simulink model "Stateflows"  (R2020a)
settings: Solver=FixedStepAuto  StartTime=0.0  StopTime=10.0  FixedStep=1e-3  RelTol=1e-3  EnableMultiTasking=on
undefined symbols (not defined in the file): D0, D1, D10, D11, D12, D13, D2, D3, D4, D5, D6, D7, D8, D9, PTA0, PTA1, PTA2, PTB23, PTB9, PTC16, PTC17, PTC2, PTC3, PTC4, PTD0, PTD1, PTD2, PTD3
libraries: frdmk64flib x17
settings Model: ExtModeTrigDuration=5  Creator=Luis  LastModifiedBy=jordanbierbrier
settings OptimizationCC: EnhancedBackFolding=on  PassReuseOutputArgsAs=Individual arguments  ZeroExternalMemoryAtStartup=off  ZeroInternalMemoryAtStartup=off  MaxStackSize=64  OptimizeBlockOrder=speed  DifferentSizesBufferReuse=on  OptimizationCustomize=off  EfficientTunableParamExpr=on
settings DebuggingCC: ParameterTunabilityLossMsg=error
settings HardwareCC: ProdBitPerPointer=32  ProdBitPerSizeT=32  ProdBitPerPtrDiffT=32  ProdLargestAtomicInteger=Long  ProdLargestAtomicFloat=Double  ProdWordSize=32  ProdHWDeviceType=ARM Compatible->ARM Cortex
settings SFSimCC: MATLABDynamicMemAlloc=off
settings RTWCC: SystemTargetFile=ert.tlc  HardwareBoard=NXP FRDM-K64F  TemplateMakefile=ert_default_tmf  Toolchain=GNU Tools for ARM Embedded Processors
settings CodeAppCC: ForceParamTrailComments=on  IgnoreCustomStorageClasses=off  OperatorAnnotations=on  SimulinkDataObjDesc=on  SFDataObjDesc=on  InsertBlockDesc=on

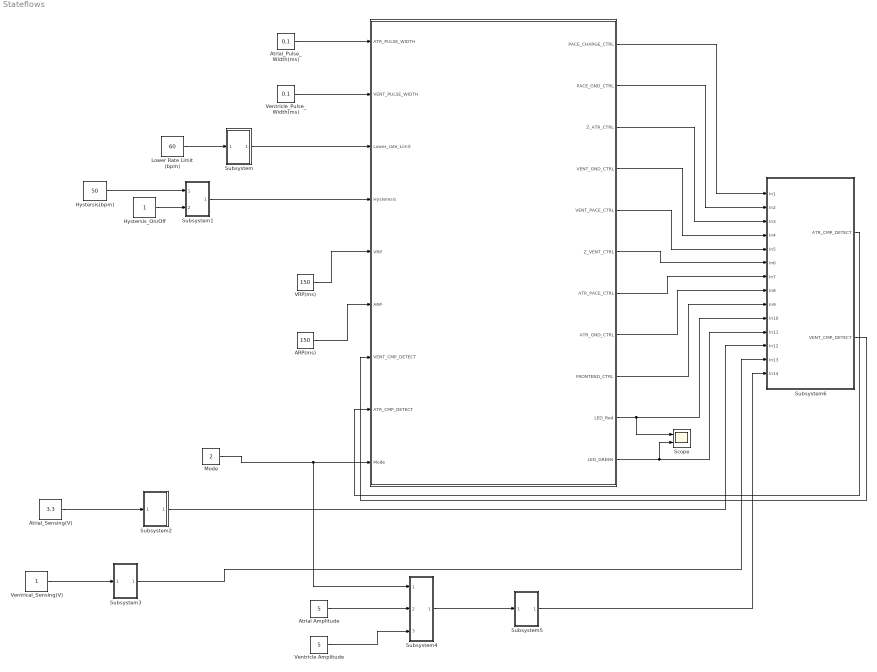
== system Stateflows ==
  " " : Stateflow chart  TreatAsAtomicUnit=on
      settings: PortSchema="{\"entries\":[{\"content\":{\"sides\":[{\"content\":{\"connectorIds\":[\"In1\",\"In4\",\"In2\",\"In9\",\"In5\",\"In6\",\"In7\",\"In8\",\"In3\"]},\"type\":\"ConnectorPlacement.EquallySpacedRectSide\",\"uuid\":\"f97b12ff-cb00-4386-a373-7143c3a8b48d\"},{\"content\":{\"connectorIds\":[\"Out1\",\"Out2\",\"Out3\",\"Out4\",\"Out5\",\"Out6\",\"Out7\",\"Out8\",\"Out9\",\"Out10\",\"Out11\"],\"side\":\"RIGHT\"},\"type\":\"ConnectorPlacement.EquallySpacedRectSide\",\"uuid\":\"90163773-f9d1-46de-bd72-9589b8539202\"},{\"content\":{\"connectorIds\":[],\"side\":\"TOP\"},\"type\":\"ConnectorPlacement.EquallySpacedRectSide\",\"uuid\":\"f8a54119-a7c4-4071-8260-df405210e670\"}]},\"type\":\"ConnectorPlacement.EquallySpacedConnector\",\"uuid\":\"47f7c40c-c42b-42f7-beed-99d299c6cdee\"}],\"packageUris\":[\"http://schema.mathworks.com/mf0/Connector/19700101\"],\"version\":\"1.0\"}"
  ARP(ms) : Constant  Value=150  OutDataTypeStr=uint16
  Atrial Amplitude : Constant  Value=5  OutDataTypeStr=double
  Atrial_Pulse_Width(ms) : Constant  Value=0.1  OutDataTypeStr=double
  Atrial_Sensing(V) : Constant  Value=3.3  OutDataTypeStr=double
  Hystersis(bpm) : Constant  Value=50  OutDataTypeStr=uint16
  Hystersis_On/Off : Constant  OutDataTypeStr=uint16
  Lower Rate Limit (bpm) : Constant  Value=60  OutDataTypeStr=uint16
  Mode : Constant  Value=2  OutDataTypeStr=uint8
  Scope : Scope  NumInputPorts=2
  Subsystem : Subsystem
  Subsystem1 : Subsystem
  Subsystem2 : Subsystem
  Subsystem3 : Subsystem
  Subsystem4 : Subsystem
  Subsystem5 : Subsystem
  Subsystem6 : Subsystem
  VRP(ms) : Constant  Value=150  OutDataTypeStr=uint16
  Ventrical_Sensing(V) : Constant  OutDataTypeStr=double
  Ventricle Amplitude : Constant  Value=5  OutDataTypeStr=double
  Ventricle_Pulse_Width(ms) : Constant  Value=0.1  OutDataTypeStr=double
  wires:
  Atrial_Pulse_Width(ms)/1 -> " "/1(ATR_PULSE_WIDTH)
  Mode/1 -> Subsystem4/1(In1), " "/3(Mode)
  Ventricle_Pulse_Width(ms)/1 -> " "/4(VENT_PULSE_WIDTH)
  ARP(ms)/1 -> " "/6(ARP)
  VRP(ms)/1 -> " "/5(VRP)
  Lower Rate Limit (bpm)/1 -> Subsystem/1(In1)
  Subsystem/1(Out1) -> " "/2(Lower_rate_Limit)
  Hystersis(bpm)/1 -> Subsystem1/1(In1)
  Hystersis_On/Off/1 -> Subsystem1/2(In2)
  Subsystem1/1(Out1) -> " "/9(Hysteresis)
  Atrial_Sensing(V)/1 -> Subsystem2/1(In1)
  Ventrical_Sensing(V)/1 -> Subsystem3/1(In1)
  Atrial Amplitude/1 -> Subsystem4/2(In2)
  Ventricle Amplitude/1 -> Subsystem4/3(In3)
  Subsystem4/1(Out1) -> Subsystem5/1(In1)
  " "/1(PACE_CHARGE_CTRL) -> Subsystem6/1(In1)
  " "/2(PACE_GND_CTRL) -> Subsystem6/2(In2)
  " "/3(Z_ATR_CTRL) -> Subsystem6/3(In3)
  " "/4(VENT_GND_CTRL) -> Subsystem6/4(In4)
  " "/5(VENT_PACE_CTRL) -> Subsystem6/5(In5)
  " "/6(Z_VENT_CTRL) -> Subsystem6/6(In6)
  " "/7(ATR_PACE_CTRL) -> Subsystem6/7(In7)
  " "/8(ATR_GND_CTRL) -> Subsystem6/8(In8)
  " "/9(FRONTEND_CTRL) -> Subsystem6/9(In9)
  " "/10(LED_Red) -> Scope/1, Subsystem6/10(In10)
  " "/11(LED_GREEN) -> Scope/2, Subsystem6/11(In11)
  Subsystem2/1(Out1) -> Subsystem6/12(In12)
  Subsystem3/1(Out1) -> Subsystem6/13(In13)
  Subsystem5/1(Out1) -> Subsystem6/14(In14)
  Subsystem6/1(ATR_CMP_DETECT) -> " "/8(ATR_CMP_DETECT)
  Subsystem6/2(VENT_CMP_DETECT) -> " "/7(VENT_CMP_DETECT)

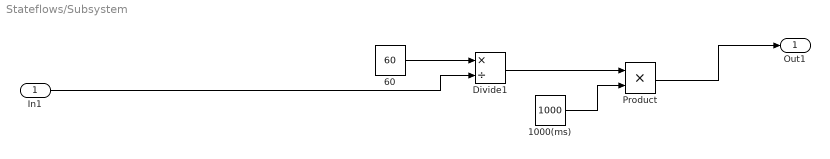
== system Stateflows/Subsystem ==
  In1 : Inport
  1000(ms) : Constant  Value=1000  OutDataTypeStr=uint16
  60 : Constant  Value=60  OutDataTypeStr=uint16
  Divide1 : Product  Inputs=*/
  Product : Product  OutDataTypeStr=uint16
  Out1 : Outport
  wires:
  60/1 -> Divide1/1
  In1/1 -> Divide1/2
  Product/1 -> Out1/1
  Divide1/1 -> Product/1
  1000(ms)/1 -> Product/2

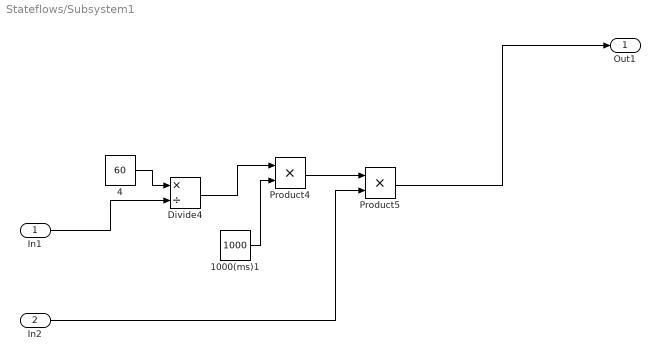
== system Stateflows/Subsystem1 ==
  In1 : Inport
  In2 : Inport  Port=2
  1000(ms)1 : Constant  Value=1000  OutDataTypeStr=uint16
  4 : Constant  Value=60  OutDataTypeStr=uint16
  Divide4 : Product  Inputs=*/
  Product4 : Product  OutDataTypeStr=uint16
  Product5 : Product  OutDataTypeStr=uint16
  Out1 : Outport
  wires:
  In2/1 -> Product5/2
  Product5/1 -> Out1/1
  Divide4/1 -> Product4/1
  Product4/1 -> Product5/1
  4/1 -> Divide4/1
  In1/1 -> Divide4/2
  1000(ms)1/1 -> Product4/2

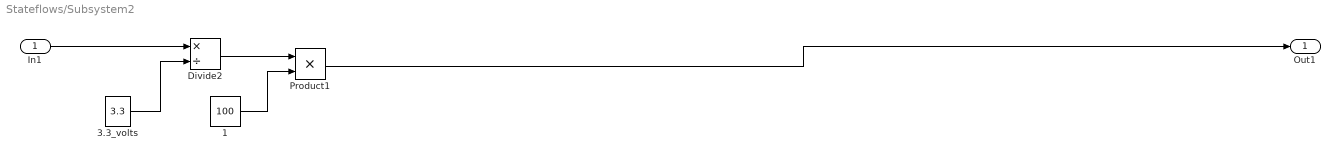
== system Stateflows/Subsystem2 ==
  In1 : Inport
  1 : Constant  Value=100  OutDataTypeStr=uint16
  3.3_volts : Constant  Value=3.3  OutDataTypeStr=double
  Divide2 : Product  Inputs=*/
  Product1 : Product  OutDataTypeStr=uint16
  Out1 : Outport
  wires:
  Product1/1 -> Out1/1
  1/1 -> Product1/2
  In1/1 -> Divide2/1
  Divide2/1 -> Product1/1
  3.3_volts/1 -> Divide2/2

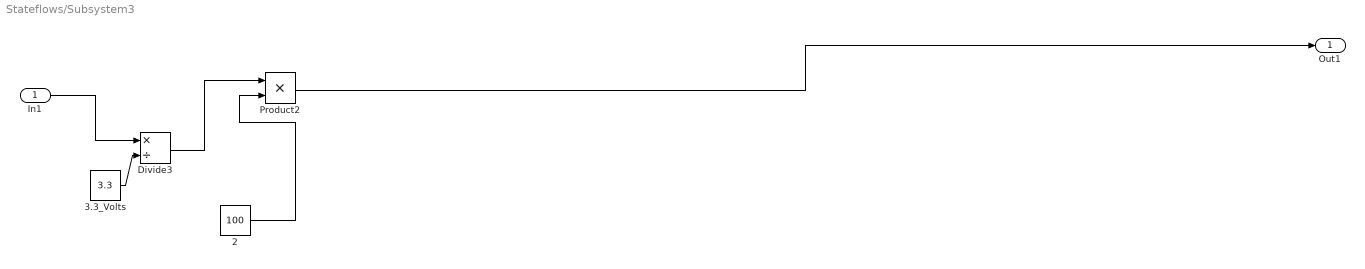
== system Stateflows/Subsystem3 ==
  In1 : Inport
  2 : Constant  Value=100  OutDataTypeStr=uint16
  3.3_Volts : Constant  Value=3.3  OutDataTypeStr=double
  Divide3 : Product  Inputs=*/
  Product2 : Product  OutDataTypeStr=uint16
  Out1 : Outport
  wires:
  Product2/1 -> Out1/1
  3.3_Volts/1 -> Divide3/2
  Divide3/1 -> Product2/1
  In1/1 -> Divide3/1
  2/1 -> Product2/2

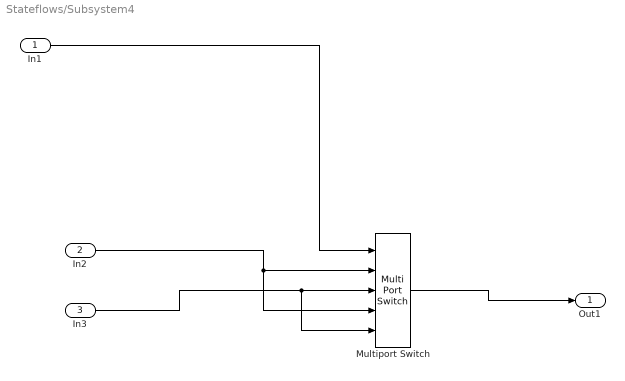
== system Stateflows/Subsystem4 ==
  In1 : Inport
  In2 : Inport  Port=2
  In3 : Inport  Port=3
  Multiport Switch : MultiPortSwitch  DataPortOrder=Zero-based contiguous  Inputs=4  zeroidx=on  OutDataTypeStr=double
  Out1 : Outport
  wires:
  Multiport Switch/1 -> Out1/1
  In3/1 -> Multiport Switch/5, Multiport Switch/3
  In1/1 -> Multiport Switch/1
  In2/1 -> Multiport Switch/4, Multiport Switch/2

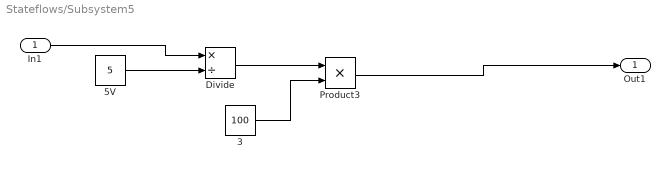
== system Stateflows/Subsystem5 ==
  In1 : Inport
  3 : Constant  Value=100  OutDataTypeStr=uint16
  5V : Constant  Value=5  OutDataTypeStr=uint16
  Divide : Product  Inputs=*/  OutDataTypeStr=uint16
  Product3 : Product  OutDataTypeStr=uint16
  Out1 : Outport
  wires:
  Product3/1 -> Out1/1
  3/1 -> Product3/2
  In1/1 -> Divide/1
  Divide/1 -> Product3/1
  5V/1 -> Divide/2

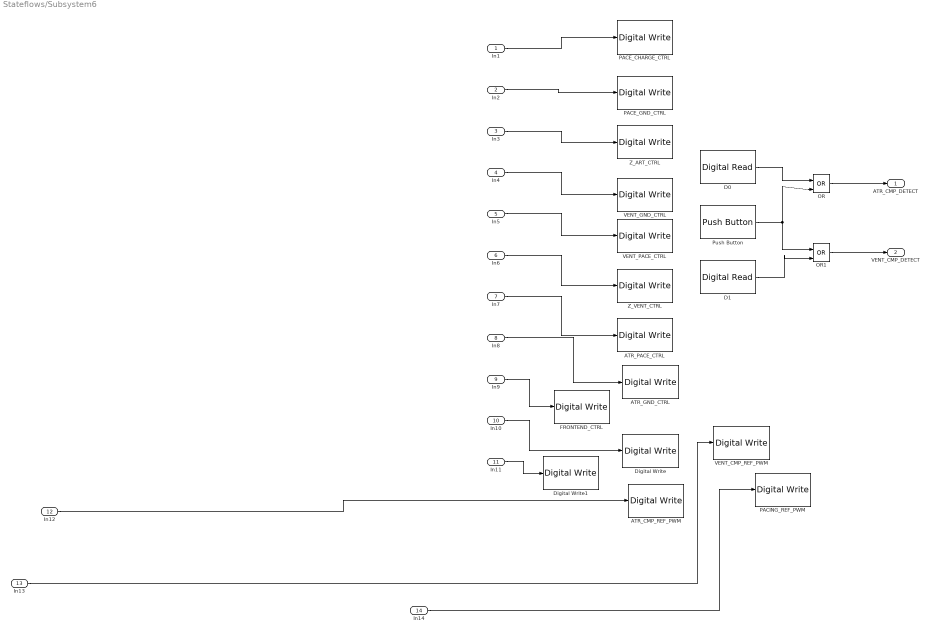
== system Stateflows/Subsystem6 ==
  In1 : Inport
  In2 : Inport  Port=2
  In3 : Inport  Port=3
  In4 : Inport  Port=4
  In5 : Inport  Port=5
  In6 : Inport  Port=6
  In7 : Inport  Port=7
  In8 : Inport  Port=8
  In9 : Inport  Port=9
  In10 : Inport  Port=10
  In11 : Inport  Port=11
  In12 : Inport  Port=12
  In13 : Inport  Port=13
  In14 : Inport  Port=14
  ATR_CMP_REF_PWM : frdmk64flib/Digital Write  Whichpin=PTC2 (D6)
  ATR_GND_CTRL : frdmk64flib/Digital Write  Whichpin=PTD2 (D11)
  ATR_PACE_CTRL : frdmk64flib/Digital Write  Whichpin=PTA0 (D8)
  D0 : frdmk64flib/Digital Read  Whichpin=PTC16 (D0)  SampleTime=-1
  D1 : frdmk64flib/Digital Read  Whichpin=PTC17 (D1)  SampleTime=-1
  Digital Write : frdmk64flib/Digital Write  Whichpin=RED_LED
  Digital Write1 : frdmk64flib/Digital Write  Whichpin=GREEN_LED
  FRONTEND_CTRL : frdmk64flib/Digital Write  Whichpin=PTD1 (D13)
  OR : Logic  Operator=OR  IconShape=distinctive  AllPortsSameDT=off  OutDataTypeStr=boolean
  OR1 : Logic  Operator=OR  IconShape=distinctive  AllPortsSameDT=off  OutDataTypeStr=boolean
  PACE_CHARGE_CTRL : frdmk64flib/Digital Write  Whichpin=PTB9 (D2)
  PACE_GND_CTRL : frdmk64flib/Digital Write  Whichpin=PTD0 (D10)
  PACING_REF_PWM : frdmk64flib/Digital Write  Whichpin=PTA2 (D5)
  Push Button : frdmk64flib/Push Button  Whichswitch=SW2  SampleTime1=-1
  VENT_CMP_REF_PWM : frdmk64flib/Digital Write  Whichpin=PTA1 (D3)
  VENT_GND_CTRL : frdmk64flib/Digital Write  Whichpin=PTD3 (D12)
  VENT_PACE_CTRL : frdmk64flib/Digital Write  Whichpin=PTC4 (D9)
  Z_ART_CTRL : frdmk64flib/Digital Write  Whichpin=PTB23 (D4)
  Z_VENT_CTRL : frdmk64flib/Digital Write  Whichpin=PTC3 (D7)
  ATR_CMP_DETECT : Outport
  VENT_CMP_DETECT : Outport  Port=2
  wires:
  In14/1 -> PACING_REF_PWM/1
  In10/1 -> Digital Write/1
  In3/1 -> Z_ART_CTRL/1
  In1/1 -> PACE_CHARGE_CTRL/1
  In4/1 -> VENT_GND_CTRL/1
  D1/1 -> OR1/2
  In7/1 -> ATR_PACE_CTRL/1
  OR1/1 -> VENT_CMP_DETECT/1
  In2/1 -> PACE_GND_CTRL/1
  In8/1 -> ATR_GND_CTRL/1
  OR/1 -> ATR_CMP_DETECT/1
  D0/1 -> OR/1
  In12/1 -> ATR_CMP_REF_PWM/1
  Push Button/1 -> OR1/1, OR/2
  In11/1 -> Digital Write1/1
  In9/1 -> FRONTEND_CTRL/1
  In13/1 -> VENT_CMP_REF_PWM/1
  In6/1 -> Z_VENT_CTRL/1
  In5/1 -> VENT_PACE_CTRL/1

== stateflow chart Stateflows/  ==
  state AOO
    state AOO_CHARGING
      entry:
      %Charge C22
      ATR_PACE_CTRL=false;
      VENT_PACE_CTRL=false;
      PACE_CHARGE_CTRL=true;
      %Discharge C21
      PACE_GND_CTRL=true;
      Z_VENT_CTRL=false;
      Z_ATR_CTRL=false;
      ATR_GND_CTRL=true;
      VENT_GND_CTRL=false;
      LED_Red = false;
    state AOO_DISCHARGING
      entry:
      %Discharge C22 into ATR
      %Charge C21
      PACE_CHARGE_CTRL=false;
      PACE_GND_CTRL=true;
      ATR_PACE_CTRL=true;
      ATR_GND_CTRL=false;
      Z_VENT_CTRL=false;
      Z_ATR_CTRL=false;
      VENT_GND_CTRL=false;
      VENT_PACE_CTRL=false;
      LED_Red = true;
    AOO_DISCHARGING -> AOO_CHARGING : after(ATR_PULSE_WIDTH,msec)
    AOO_CHARGING -> AOO_DISCHARGING : after(Lower_rate_Limit - ATR_PULSE_WIDTH,msec)
  state VOO [group]
    state VOO_CHARGING
      entry:
      %Charge C22
      VENT_PACE_CTRL=false;
      ATR_PACE_CTRL=false;
      PACE_CHARGE_CTRL=true;
      %Discharge C21
      PACE_GND_CTRL=true;
      Z_VENT_CTRL=false;
      Z_ATR_CTRL=false;
      ATR_PACE_CTRL=false;
      ATR_GND_CTRL=false;
      VENT_GND_CTRL=true;
      LED_GREEN = false;
    state VOO_DISCHARGE
      entry:
      %Discharge C22 into VENT
      %Charge C21
      PACE_CHARGE_CTRL=false;
      PACE_GND_CTRL=true;
      ATR_PACE_CTRL=false;
      ATR_GND_CTRL=false;
      Z_ATR_CTRL=false
      Z_VENT_CTRL=false;
      VENT_GND_CTRL=false;
      VENT_PACE_CTRL=true;
      LED_GREEN = true;
    VOO_DISCHARGE -> VOO_CHARGING : after(VENT_PULSE_WIDTH, msec)
    VOO_CHARGING -> VOO_DISCHARGE : after(Lower_rate_Limit - VENT_PULSE_WIDTH, msec)
  state VVI_Hys [group]
    state CHARGING_C22
      entry:
      FRONTEND_CTRL = true;
      PACE_GND_CTRL = true;
      VENT_PACE_CTRL=false;
      ATR_PACE_CTRL=false;
      PACE_CHARGE_CTRL=true;
      Z_VENT_CTRL=false;
      Z_ATR_CTRL=false;
      ATR_GND_CTRL=false;
      VENT_GND_CTRL=true;
      LED_GREEN = false;
    state VENTRICAL_PACE
      entry:
      FRONTEND_CTRL = false;
      PACE_GND_CTRL = true;
      VENT_PACE_CTRL=true;
      ATR_PACE_CTRL=false;
      PACE_CHARGE_CTRL=false;
      Z_VENT_CTRL=false;
      Z_ATR_CTRL=false;
      ATR_GND_CTRL=false;
      VENT_GND_CTRL=false;
      LED_GREEN = true;
    state VRP
      entry:
      PACE_GND_CTRL = true;
      VENT_PACE_CTRL=false;
      ATR_PACE_CTRL=false;
      PACE_CHARGE_CTRL=true;
      Z_VENT_CTRL=false;
      Z_ATR_CTRL=false;
      ATR_GND_CTRL=false;
      VENT_GND_CTRL=true;
      LED_GREEN = false;
    VVI_Hys.CHARGING_C22 -> VVI_Hys.VENTRICAL_PACE [order 2] : after((Lower_rate_Limit - VENT_PULSE_WIDTH - VRP + Hysteresis - Lower_rate_Limit), msec)
    VVI_Hys.CHARGING_C22 -> VVI_Hys.VRP [order 1] : [VENT_CMP_DETECT == true]
    VVI_Hys.VRP -> VVI_Hys.CHARGING_C22 : after(VRP, msec)
    VVI_Hys.VENTRICAL_PACE -> VVI_Hys.VRP : after(VENT_PULSE_WIDTH, msec)
  state Intial_State
    entry:
    %Charge C22
    ATR_PACE_CTRL=false;
    VENT_PACE_CTRL=false;
    PACE_CHARGE_CTRL=false;
    %Discharge C21
    PACE_GND_CTRL=false;
    Z_VENT_CTRL=false;
    Z_ATR_CTRL=false;
    ATR_GND_CTRL=false;
    VENT_GND_CTRL=false;
  state VVI [group]
    state CHARGING_C22
      entry:
      FRONTEND_CTRL = true;
      PACE_GND_CTRL = true;
      VENT_PACE_CTRL=false;
      ATR_PACE_CTRL=false;
      PACE_CHARGE_CTRL=true;
      Z_VENT_CTRL=false;
      Z_ATR_CTRL=false;
      ATR_GND_CTRL=false;
      VENT_GND_CTRL=true;
      LED_GREEN = false;
    state VENTRICAL_PACE
      entry:
      FRONTEND_CTRL = false;
      PACE_GND_CTRL = true;
      VENT_PACE_CTRL=true;
      ATR_PACE_CTRL=false;
      PACE_CHARGE_CTRL=false;
      Z_VENT_CTRL=false;
      Z_ATR_CTRL=false;
      ATR_GND_CTRL=false;
      VENT_GND_CTRL=false;
      LED_GREEN = true;
    state VRP
      entry:
      PACE_GND_CTRL = true;
      VENT_PACE_CTRL=false;
      ATR_PACE_CTRL=false;
      PACE_CHARGE_CTRL=true;
      Z_VENT_CTRL=false;
      Z_ATR_CTRL=false;
      ATR_GND_CTRL=false;
      VENT_GND_CTRL=true;
      LED_GREEN = false;
    VVI.CHARGING_C22 -> VVI.VENTRICAL_PACE [order 2] : after((Lower_rate_Limit - VENT_PULSE_WIDTH - VRP), msec)
    VVI.CHARGING_C22 -> VVI.VRP [order 1] : [VENT_CMP_DETECT == true]
    VVI.VRP -> VVI.CHARGING_C22 : after(VRP, msec)
    VVI.VENTRICAL_PACE -> VVI.VRP : after(VENT_PULSE_WIDTH, msec)
  state AAI [group]
    state CHARGING_C22
      entry:
      FRONTEND_CTRL = true;
      PACE_GND_CTRL = true;
      VENT_PACE_CTRL=false;
      ATR_PACE_CTRL=false;
      PACE_CHARGE_CTRL=true;
      Z_VENT_CTRL=false;
      Z_ATR_CTRL=false;
      ATR_GND_CTRL=true;
      VENT_GND_CTRL=false;
      LED_Red = false;
    state ATRIAL_PACE
      entry:
      FRONTEND_CTRL = false;
      PACE_GND_CTRL = true;
      VENT_PACE_CTRL=false;
      ATR_PACE_CTRL=true;
      PACE_CHARGE_CTRL=false;
      Z_VENT_CTRL=false;
      Z_ATR_CTRL=false;
      ATR_GND_CTRL=false;
      VENT_GND_CTRL=false;
      LED_Red = true;
    state ARP
      entry:
      PACE_GND_CTRL = true;
      VENT_PACE_CTRL=false;
      ATR_PACE_CTRL=false;
      PACE_CHARGE_CTRL=true;
      Z_VENT_CTRL=false;
      Z_ATR_CTRL=false;
      ATR_GND_CTRL=true;
      VENT_GND_CTRL=false;
      LED_Red = false;
    AAI.CHARGING_C22 -> AAI.ATRIAL_PACE [order 2] : after(Lower_rate_Limit - ATR_PULSE_WIDTH - ARP, msec)
    AAI.CHARGING_C22 -> AAI.ARP [order 1] : [ATR_CMP_DETECT == true]
    AAI.ARP -> AAI.CHARGING_C22 : after(ARP, msec)
    AAI.ATRIAL_PACE -> AAI.ARP : after(ATR_PULSE_WIDTH, msec)
  state AAI_Hys [group]
    state CHARGING_C22
      entry:
      FRONTEND_CTRL = true;
      PACE_GND_CTRL = true;
      VENT_PACE_CTRL=false;
      ATR_PACE_CTRL=false;
      PACE_CHARGE_CTRL=true;
      Z_VENT_CTRL=false;
      Z_ATR_CTRL=false;
      ATR_GND_CTRL=true;
      VENT_GND_CTRL=false;
      LED_Red = false;
    state ATRIAL_PACE
      entry:
      FRONTEND_CTRL = false;
      PACE_GND_CTRL = true;
      VENT_PACE_CTRL=false;
      ATR_PACE_CTRL=true;
      PACE_CHARGE_CTRL=false;
      Z_VENT_CTRL=false;
      Z_ATR_CTRL=false;
      ATR_GND_CTRL=false;
      VENT_GND_CTRL=false;
      LED_Red = true;
    state ARP
      entry:
      PACE_GND_CTRL = true;
      VENT_PACE_CTRL=false;
      ATR_PACE_CTRL=false;
      PACE_CHARGE_CTRL=true;
      Z_VENT_CTRL=false;
      Z_ATR_CTRL=false;
      ATR_GND_CTRL=true;
      VENT_GND_CTRL=false;
      LED_Red = false
    AAI_Hys.CHARGING_C22 -> AAI_Hys.ATRIAL_PACE [order 2] : after((Lower_rate_Limit - VENT_PULSE_WIDTH - VRP + Hysteresis - Lower_rate_Limit), msec)
    AAI_Hys.CHARGING_C22 -> AAI_Hys.ARP [order 1] : [ATR_CMP_DETECT == true]
    AAI_Hys.ARP -> AAI_Hys.CHARGING_C22 : after(ARP, msec)
    AAI_Hys.ATRIAL_PACE -> AAI_Hys.ARP : after(ATR_PULSE_WIDTH, msec)
  Intial_State -> AOO_CHARGING [order 1] : [Mode == 0]
  Intial_State -> VVI_Hys.CHARGING_C22 [order 6] : [Mode == 2 & Hysteresis > 0]
  Intial_State -> VOO_CHARGING [order 2] : [Mode == 1]
  (default) -> Intial_State
  Intial_State -> AAI_Hys.CHARGING_C22 [order 5] : [Mode == 3 & Hysteresis >0]
  Intial_State -> VVI.CHARGING_C22 [order 3] : [Mode == 2 & Hysteresis ==0]
  Intial_State -> AAI.CHARGING_C22 [order 4] : [Mode == 3 & Hysteresis == 0]
  data: PACE_CHARGE_CTRL output boolean; PACE_GND_CTRL output boolean; Z_ATR_CTRL output boolean; VENT_GND_CTRL output boolean; VENT_PACE_CTRL output boolean; Z_VENT_CTRL output boolean; ATR_PULSE_WIDTH input double; Lower_rate_Limit input uint16; Mode input uint8; ATR_PACE_CTRL output boolean; ATR_GND_CTRL output boolean; VENT_PULSE_WIDTH input double; VRP input uint16; ARP input uint16; FRONTEND_CTRL output boolean; VENT_CMP_DETECT input boolean; ATR_CMP_DETECT input boolean; LED_Red output boolean; LED_GREEN output boolean; Hysteresis input uint16
